simulink model "Ventilator_Controller"  (R2019b)
settings: Solver=ode23tb  StartTime=0  StopTime=1000  FixedStep=0.001  MaxStep=time_step_new  RelTol=0.01  EnableMultiTasking=on
values from neighbouring files (symbols this model uses):
  A = 20.9    [Gas_Exchange_IC.m]    (also in getPneumonia.m = (LF1-LF2)/(1-exp(Rresolve*(t2(end)-t2(1)))))
  a1 = 0.3836    [Dissociation_Spencer_IC.m]    (also in Gas_Exchange_IC.m; Respiratory_IC.m)
  a2 = 1.819    [Dissociation_Spencer_IC.m]    (also in Gas_Exchange_IC.m; Respiratory_IC.m)
  alpha1 = 0.02598    [Dissociation_Spencer_IC.m]    (also in Gas_Exchange_IC.m; Respiratory_IC.m)
  alpha2 = 0.05591    [Dissociation_Spencer_IC.m]    (also in Gas_Exchange_IC.m; Respiratory_IC.m)
  B = 92.8    [Gas_Exchange_IC.m]    (also in getPneumonia.m = LungFunction(end)-A)
  beta1 = 0.012275    [Dissociation_Spencer_IC.m]    (also in Gas_Exchange_IC.m; Respiratory_IC.m)
  beta2 = 0.03255    [Dissociation_Spencer_IC.m]    (also in Gas_Exchange_IC.m; Respiratory_IC.m)
  C = 10570    [Gas_Exchange_IC.m]
  C1 = 9    [Dissociation_Spencer_IC.m]    (also in Gas_Exchange_IC.m; Respiratory_IC.m)
  C2 = 87.00    (= 87)    [Dissociation_Spencer_IC.m]    (also in Gas_Exchange_IC.m; Respiratory_IC.m)
  Circadian_Period = 24    [Respiratory_IC.m]    (also in State_UA_Khoo_IC.m)
  CvCO2IC = 0.5116    [Body_Khoo_IC.m]    (also in Gas_Exchange_IC.m; Respiratory_IC.m = 0.5247)
  CvO2IC = 0.1672    [Body_Khoo_IC.m]    (also in Gas_Exchange_IC.m; Respiratory_IC.m = 0.1639)
  D = -5.251    [Gas_Exchange_IC.m]
  Dead1CO2IC = 0.1020    (= 0.102)    [Dead_Space_Khoo_IC.m]    (also in Gas_Exchange_IC.m; Respiratory_IC.m = 39.5616)
  Dead1O2IC = 149.8824    [Dead_Space_Khoo_IC.m]    (also in Gas_Exchange_IC.m; Respiratory_IC.m = 104.3637)
  Dead2CO2IC = 0.5274    [Dead_Space_Khoo_IC.m]    (also in Gas_Exchange_IC.m; Respiratory_IC.m = 39.6736)
  Dead2O2IC = 149.3923    [Dead_Space_Khoo_IC.m]    (also in Gas_Exchange_IC.m; Respiratory_IC.m = 104.2258)
  Dead3CO2IC = 2.2996    [Dead_Space_Khoo_IC.m]    (also in Gas_Exchange_IC.m; Respiratory_IC.m = 39.8127)
  Dead3O2IC = 147.3503    [Dead_Space_Khoo_IC.m]    (also in Gas_Exchange_IC.m; Respiratory_IC.m = 104.0505)
  Dead4CO2IC = 8.2293    [Dead_Space_Khoo_IC.m]    (also in Gas_Exchange_IC.m; Respiratory_IC.m = 40.0061)
  Dead4O2IC = 140.5179    [Dead_Space_Khoo_IC.m]    (also in Gas_Exchange_IC.m; Respiratory_IC.m = 103.8005)
  Dead5CO2IC = 22.0757    [Dead_Space_Khoo_IC.m]    (also in Gas_Exchange_IC.m; Respiratory_IC.m = 40.3359)
  Dead5O2IC = 124.5641    [Dead_Space_Khoo_IC.m]    (also in Gas_Exchange_IC.m; Respiratory_IC.m = 103.3579)
  DtotalIC = 0.3    [NeuroMuscular_IC.m]    (also in Respiratory_IC.m = 0.32)
  E_CW = 5    [Pleural_Schuessler_IC.m]    (also in Pmus_Flow_Younes_IC.m; Resp_Mech_IC.m; Respiratory_IC.m)
  E_L = 5    [Pleural_Schuessler_IC.m]    (also in Pmus_Flow_Younes_IC.m; Resp_Mech_IC.m; Respiratory_IC.m)
  fc = 0.4/60    (= 0.00666666666667)    [Respiratory_IC.m]    (also in State_UA_Khoo_IC.m)
  fcs_max = 47.78    [Cardiovascular_IC.m]    (also in Reflex_Ursino_IC.m)
  fcs_min = 2.52    [Cardiovascular_IC.m]    (also in Reflex_Ursino_IC.m)
  fcs_zero = 25    [Respiratory_IC.m]
  FlowIC = 0    [Pmus_Flow_Younes_IC.m]    (also in Resp_Mech_IC.m; Respiratory_IC.m)
  fp_inf = 6.3    [Respiratory_IC.m]
  fp_zero = 3.2    [Respiratory_IC.m]
  fs_inf = 2.10    (= 2.1)    [Respiratory_IC.m]
  fs_zero = 16.11    [Respiratory_IC.m]
  ftbs_min = 0.1    [Cardiovascular_IC.m]    (also in SA_Node_Ursino_IC.m)
  gc = 0.008/60    (= 0.000133333333333)    [Respiratory_IC.m]    (also in State_UA_Khoo_IC.m)
  h = 0.0183    [Brain_Khoo_IC.m]    (also in Gas_Exchange_IC.m; Respiratory_IC.m)
  HP_basal = 0.58    [Cardiovascular_IC.m]    (also in SA_Node_Ursino_IC.m)
  Ic = 45    [Gas_Exchange_IC.m]    (also in Respiratory_IC.m; Vent_Drive_Khoo_IC.m)
  IpCO2 = 38    [Gas_Exchange_IC.m]    (also in Respiratory_IC.m; Vent_Drive_Khoo_IC.m)
  IpO2 = 102.4    [Gas_Exchange_IC.m]    (also in Respiratory_IC.m; Vent_Drive_Khoo_IC.m)
  K1 = 13    [Dissociation_Spencer_IC.m]    (also in Gas_Exchange_IC.m; Respiratory_IC.m)
  K2 = 194.4    [Dissociation_Spencer_IC.m]    (also in Gas_Exchange_IC.m; Respiratory_IC.m)
  k_cs = 11.758    [Cardiovascular_IC.m]    (also in Reflex_Ursino_IC.m)
  k_p = 7.06    [Respiratory_IC.m]
  k_s = 0.07    [Respiratory_IC.m]
  lambda = 863    [Gas_Exchange_IC.m]    (also in Lungs_Khoo_IC.m; Respiratory_IC.m)
  Mech_Vent_pressure = 17    [Mech_vent_test.m]
  MRbCO2 = 0.0517    [Brain_Khoo_IC.m]    (also in Gas_Exchange_IC.m; Respiratory_IC.m)
  MRCO2 = 0.0033    [Body_Khoo_IC.m]    (also in Gas_Exchange_IC.m; Respiratory_IC.m)
  MRO2 = 0.0038    [Body_Khoo_IC.m]    (also in Gas_Exchange_IC.m; Respiratory_IC.m)
  NM_block_gain = 1    [Mech_vent_test.m]
  PACO2_delayIC = 39.6041    [Cardio_Mix_Lange_IC.m]    (also in Gas_Exchange_IC.m; Respiratory_IC.m = 40.4448)
  PaCO2firstIC = 0.2150    (= 0.215)    [Cardio_Mix_Lange_IC.m]    (also in Gas_Exchange_IC.m; Respiratory_IC.m = -0.2465)
  PACO2IC = 37.1484    [Gas_Exchange_IC.m]    (also in Lungs_Khoo_IC.m; Respiratory_IC.m = 40.9432)
  PaCO2secondIC = 38.4577    [Cardio_Mix_Lange_IC.m]    (also in Gas_Exchange_IC.m; Respiratory_IC.m = 40.3928)
  PAO2_delayIC = 103.8436    [Cardio_Mix_Lange_IC.m]    (also in Gas_Exchange_IC.m; Respiratory_IC.m = 103.1223)
  PaO2firstIC = -0.2838    [Cardio_Mix_Lange_IC.m]    (also in Gas_Exchange_IC.m; Respiratory_IC.m = 0.3557)
  PAO2IC = 107.1983    [Gas_Exchange_IC.m]    (also in Lungs_Khoo_IC.m; Respiratory_IC.m = 102.5153)
  PaO2secondIC = 105.4828    [Cardio_Mix_Lange_IC.m]    (also in Gas_Exchange_IC.m; Respiratory_IC.m = 103.1435)
  PbCO2IC = 48.2858    [Brain_Khoo_IC.m]    (also in Gas_Exchange_IC.m; Respiratory_IC.m = 48.5383)
  PICO2 = 0    [Dead_Space_Khoo_IC.m]    (also in Gas_Exchange_IC.m; Respiratory_IC.m)
  PICO2_change = 0    [Respiratory_IC.m]
  PIO2 = 150    [Dead_Space_Khoo_IC.m]    (also in Gas_Exchange_IC.m; Respiratory_IC.m)
  PIO2_change = -90    [Mech_vent_test.m]    (also in Respiratory_IC.m = 0)
  Pn = 90    [Cardiovascular_IC.m]    (also in Reflex_Ursino_IC.m)
  Pt_frcIC1 = 0    [Pmus_Flow_Younes_IC.m]    (also in Resp_Mech_IC.m; Respiratory_IC.m)
  Pt_frcIC2 = 0    [Pmus_Flow_Younes_IC.m]    (also in Resp_Mech_IC.m; Respiratory_IC.m)
  QdBo = 0.8333    [Brain_Khoo_IC.m]    (also in Gas_Exchange_IC.m; Respiratory_IC.m)
  R_AW = 1.27    [Pleural_Schuessler_IC.m]    (also in Pmus_Flow_Younes_IC.m; Resp_Mech_IC.m; Respiratory_IC.m)
  R_CW = 1.03    [Pleural_Schuessler_IC.m]    (also in Pmus_Flow_Younes_IC.m; Resp_Mech_IC.m; Respiratory_IC.m)
  R_L = 1.69    [Pleural_Schuessler_IC.m]    (also in Pmus_Flow_Younes_IC.m; Resp_Mech_IC.m; Respiratory_IC.m)
  RC = 0.06    [Pleural_Schuessler_IC.m]    (also in Pmus_Flow_Younes_IC.m; Resp_Mech_IC.m; Respiratory_IC.m)
  rc = 0.2/60    (= 0.00333333333333)    [Respiratory_IC.m]    (also in State_UA_Khoo_IC.m)
  SbCO2 = 0.3600    (= 0.36)    [Brain_Khoo_IC.m]    (also in Gas_Exchange_IC.m; Respiratory_IC.m)
  SCO2 = 0.0043    [Brain_Khoo_IC.m]    (also in Gas_Exchange_IC.m; Respiratory_IC.m)
  SWAo = 0.007    [Respiratory_IC.m]    (also in State_UA_Khoo_IC.m)
  T1 = 1    [Cardio_Mix_Lange_IC.m]    (also in Gas_Exchange_IC.m; Respiratory_IC.m)
  T2 = 2    [Cardio_Mix_Lange_IC.m]    (also in Gas_Exchange_IC.m; Respiratory_IC.m)
  t_CO2_duration = 0    [Respiratory_IC.m]
  t_CO2_start = 0    [Respiratory_IC.m]
  t_end_new = 4*24*60*60    (= 345600)    [Mech_vent_test.m]
  t_end_UA = 0    [Respiratory_IC.m]    (also in State_UA_Khoo_IC.m)
  t_Mech_Vent_duration = 0    [Mech_vent_test.m]
  t_Mech_Vent_start = 0    [Mech_vent_test.m]
  t_Mueller_duration = 0    [NeuroMuscular_IC.m]
  t_Mueller_insp = 0    [NeuroMuscular_IC.m]
  t_Mueller_start = 0    [NeuroMuscular_IC.m]
  t_NM_block_duration = 0    [Mech_vent_test.m]
  t_NM_block_start = 0    [Mech_vent_test.m]
  t_O2_duration = 0    [Mech_vent_test.m]    (also in Respiratory_IC.m)
  t_O2_start = 0    [Mech_vent_test.m]    (also in Respiratory_IC.m)
  t_start_new = 0    [Mech_vent_test.m]
  t_start_UA = 0    [Respiratory_IC.m]    (also in State_UA_Khoo_IC.m)
  t_valsalva_duration = 0    [NeuroMuscular_IC.m]
  t_valsalva_insp = 0    [NeuroMuscular_IC.m]
  t_valsalva_start = 0    [NeuroMuscular_IC.m]
  time_step = time_step    [acquire_data.m]    (also in acquire_data_save.m)
  VC = 5    [Pmus_Flow_Younes_IC.m]    (also in Resp_Mech_IC.m; Respiratory_IC.m)
  Vdead1 = 0.03    [Dead_Space_Khoo_IC.m]    (also in Gas_Exchange_IC.m; Respiratory_IC.m)
  Vdead2 = 0.03    [Dead_Space_Khoo_IC.m]    (also in Gas_Exchange_IC.m; Respiratory_IC.m)
  Vdead3 = 0.03    [Dead_Space_Khoo_IC.m]    (also in Gas_Exchange_IC.m; Respiratory_IC.m)
  Vdead4 = 0.03    [Dead_Space_Khoo_IC.m]    (also in Gas_Exchange_IC.m; Respiratory_IC.m)
  Vdead5 = 0.03    [Dead_Space_Khoo_IC.m]    (also in Gas_Exchange_IC.m; Respiratory_IC.m)
  Ventilator_rate = 12    [Mech_vent_test.m]
  VTCO2 = 15    [Body_Khoo_IC.m]    (also in Gas_Exchange_IC.m; Respiratory_IC.m)
  VtIC = 0    [Pmus_Flow_Younes_IC.m]    (also in Resp_Mech_IC.m; Respiratory_IC.m)
  VTO2 = 6    [Body_Khoo_IC.m]    (also in Gas_Exchange_IC.m; Respiratory_IC.m)
  Z = 0.0227    [Dissociation_Spencer_IC.m]    (also in Gas_Exchange_IC.m; Respiratory_IC.m)
undefined symbols (not defined in the file or in its folder): A_0_ua, alpha_E_FFA_Heart, alpha_E_FFA_muscle, alpha_E_GLC_Heart, alpha_E_GLC_muscle, alpha_E_GLY_muscle, alpha_E_PYR_muscle, alpha_E_TGL_adipose, alpha_E_TGL_GI, alpha_E_TGL_Heart, alpha_E_TGL_muscle, Arousal_UAIC, C_ua_awake, Cbp, Cbv, Ce_0, Cep, Cev, Chp, Chv, Cla, Clamp_class, Cmp, Cmv, Cpa, CPAP_pressure, Cpp, Cpv, Cra, Csa, Csp, Csv, CvbO2_n, CvhO2_n, CvmO2_n, DAY, delay, DietBlock, Dx, Fb, fchemo_max, fchemo_min, fchemoIC, flsIC, Ftas_I0, ftas_min, ftas_r0, FVC_activation, gain_E, Gamma, Gas_sleep, Gas_sleepM, Gb, Gblock, GbO2, Gbs_sleep, gcc_sa, gcc_sb, gcc_sp, Gclamp ... (+147)
libraries: simulink x4, simulink_extras x2
(part 4 of 8)

== system Ventilator_Controller/Cardiovascular System/SA-node and Autonomic Control/Heart Emaxrv ==
  ftbs : Inport
  Gbs(SI) : Inport  Port=2
  Constant : Constant  Value=ftbs_min
  Constant1 : Constant  Value=initx(2)
  Gain_Emaxrv : Gain  Gain=0.282  SaturateOnIntegerOverflow=on  OutDataTypeStr=Inherit: Same as input  ParamDataTypeStr=Inherit: Same as input
  Math Function : Math  Operator=log  SaturateOnIntegerOverflow=on
  Product3 : Product  SaturateOnIntegerOverflow=on  InputSameDT=on  OutDataTypeStr=Inherit: Same as first input
  Saturation : Saturate  UpperLimit=inf  LowerLimit=1
  Sum : Sum  Inputs=|+-  SaturateOnIntegerOverflow=on  InputSameDT=on  OutDataTypeStr=Inherit: Same as first input
  Sum1 : Sum  SaturateOnIntegerOverflow=on  InputSameDT=on  OutDataTypeStr=Inherit: Same as first input
  Transfer Fcn : TransferFcn  Denominator=[toux(2) 1]
  Transport Delay : TransportDelay  DelayTime=Dx(2)  BufferSize=19456
  Emaxrv : Outport
  wires:
  Constant1/1 -> Sum1/2
  Sum1/1 -> Emaxrv/1
  Transfer Fcn/1 -> Sum1/1
  Math Function/1 -> Gain_Emaxrv/1
  Saturation/1 -> Math Function/1
  Sum/1 -> Saturation/1
  Constant/1 -> Sum/2
  Transport Delay/1 -> Sum/1
  ftbs/1 -> Transport Delay/1
  Gbs(SI)/1 -> Product3/2
  Gain_Emaxrv/1 -> Product3/1
  Product3/1 -> Transfer Fcn/1

== system Ventilator_Controller/Cardiovascular System/SA-node and Autonomic Control/Hypoxia or hypercapnia1 ==
  Drive : Inport
  Divide : Product  Inputs=**
  Power : Outport
  wires:
  [MuscleContractility] -> Divide/1
  Divide/1 -> Power/1  "muscle power"
  Drive/1 -> Divide/2  "Muscle drive"

== system Ventilator_Controller/Cardiovascular System/SA-node and Autonomic Control/Hypoxia or hypercapnia2 ==
  Drive : Inport
  Divide : Product  Inputs=**
  Power : Outport
  wires:
  [MuscleContractility] -> Divide/1
  Divide/1 -> Power/1  "muscle power"
  Drive/1 -> Divide/2  "Muscle drive"

== system Ventilator_Controller/Cardiovascular System/SA-node and Autonomic Control/Left Ventricle ==
  phi : Inport
  Constant13 : Constant  Value=Vulv
  Constant14 : Constant  Value=P0lv
  Constant6 : Constant
  Fcn : Fcn  Expr=exp(u*KElv)-1
  Product4 : Product  Inputs=3  SaturateOnIntegerOverflow=on  RndMeth=Zero  InputSameDT=on  OutDataTypeStr=Inherit: Same as first input
  Product5 : Product  Inputs=3  SaturateOnIntegerOverflow=on  RndMeth=Zero  InputSameDT=on  OutDataTypeStr=Inherit: Same as first input
  SubSystem1 : Subsystem
  Sum2 : Sum  SaturateOnIntegerOverflow=on  InputSameDT=on  OutDataTypeStr=Inherit: Same as first input
  Sum3 : Sum  Inputs=-+  SaturateOnIntegerOverflow=on  InputSameDT=on  OutDataTypeStr=Inherit: Same as first input
  Pmaxlv : Outport
  wires:
  Sum2/1 -> Pmaxlv/1
  Product4/1 -> Sum2/1
  Product5/1 -> Sum2/2
  Fcn/1 -> Product5/1
  Constant14/1 -> Product5/2
  Sum3/1 -> Product5/3
  Constant6/1 -> Sum3/2
  Constant13/1 -> SubSystem1/1(_)
  [Vlv] -> SubSystem1/2(+)
  SubSystem1/1(Out) -> Product4/2
  phi/1 -> Sum3/1, Product4/3
  [Emaxlv] -> Product4/1
  [Vlv] -> Fcn/1

== system Ventilator_Controller/Cardiovascular System/SA-node and Autonomic Control/RR Interval ==
  HP_SAnode : Inport
  Abs : Abs  SaturateOnIntegerOverflow=on
  Derivative1 : Derivative
  If : If  IfExpression=u1 <0  ShowElse=off
  If Action Subsystem : Subsystem  TreatAsAtomicUnit=on
  Integrator : Integrator  ExternalReset=rising  UpperSaturationLimit=10  LowerSaturationLimit=0
  Integrator1 : Integrator  ExternalReset=rising  UpperSaturationLimit=10  LowerSaturationLimit=0
  Math Function : Math  Operator=reciprocal  SaturateOnIntegerOverflow=on
  Memory : Memory
  Mux : Mux
  Saving varHeartPeriod : Subsystem
  Sign1 : Signum  ZeroCross=off
  Sum : Sum  Inputs=+-  SaturateOnIntegerOverflow=on
  Threshold Integrated HP : Constant
  Time Constant : Constant
  Heart_Period : Outport
  wires:
  Threshold Integrated HP/1 -> Sum/1
  Integrator/1 -> Sum/2
  Sum/1 -> If/1, Mux/2  "HPin"
  Memory/1 -> Integrator/2, Integrator1/2
  Sign1/1 -> Abs/1
  Derivative1/1 -> Sign1/1
  Abs/1 -> Memory/1  "Enable signal"
  HP_SAnode/1 -> Math Function/1
  Time Constant/1 -> Integrator1/1
  Integrator1/1 -> If Action Subsystem/1(In1), Mux/3  "HPout"
  If Action Subsystem/1(Out1) -> Derivative1/1, Heart_Period/1, Mux/4  "Heart Period"
  If/1 -> If Action Subsystem/Action
  Math Function/1 -> Integrator/1, Mux/1
  Mux/1 -> Saving varHeartPeriod/1(In1)

== system Ventilator_Controller/Cardiovascular System/SA-node and Autonomic Control/Right Ventricle ==
  phi : Inport
  Constant13 : Constant  Value=Vurv
  Constant14 : Constant  Value=P0rv
  Constant6 : Constant
  Fcn : Fcn  Expr=exp(u*KErv)-1
  Product4 : Product  Inputs=3  SaturateOnIntegerOverflow=on  RndMeth=Zero  InputSameDT=on  OutDataTypeStr=Inherit: Same as first input
  Product5 : Product  Inputs=3  SaturateOnIntegerOverflow=on  RndMeth=Zero  InputSameDT=on  OutDataTypeStr=Inherit: Same as first input
  SubSystem1 : Subsystem
  Sum2 : Sum  SaturateOnIntegerOverflow=on  InputSameDT=on  OutDataTypeStr=Inherit: Same as first input
  Sum3 : Sum  Inputs=-+  SaturateOnIntegerOverflow=on  InputSameDT=on  OutDataTypeStr=Inherit: Same as first input
  Pmaxrv : Outport
  wires:
  Constant6/1 -> Sum3/2
  Sum3/1 -> Product5/3
  Constant14/1 -> Product5/2
  Fcn/1 -> Product5/1
  Product5/1 -> Sum2/2
  Product4/1 -> Sum2/1
  Sum2/1 -> Pmaxrv/1
  [Emaxrv] -> Product4/1
  [Vrv] -> SubSystem1/2(+)
  Constant13/1 -> SubSystem1/1(_)
  SubSystem1/1(Out) -> Product4/2
  phi/1 -> Sum3/1, Product4/3
  [Vrv] -> Fcn/1

== system Ventilator_Controller/Cardiovascular System/SA-node and Autonomic Control/SA Node ==
  ftbs : Inport
  ftp : Inport  Port=2
  Gbs(SI) : Inport  Port=3
  Gps(SI) : Inport  Port=4
  Constant : Constant  Value=ftbs_min
  Constant1 : Constant  Value=HP_basal
  Gain_HPbs : Gain  Gain=-0.13  SaturateOnIntegerOverflow=on  OutDataTypeStr=Inherit: Same as input  ParamDataTypeStr=Inherit: Same as input
  Gain_HPpara : Gain  Gain=0.09  SaturateOnIntegerOverflow=on  OutDataTypeStr=Inherit: Same as input  ParamDataTypeStr=Inherit: Same as input
  Math Function : Math  Operator=log  SaturateOnIntegerOverflow=on
  Product1 : Product  Inputs=*/  SaturateOnIntegerOverflow=on  InputSameDT=on  OutDataTypeStr=Inherit: Same as first input
  Product3 : Product  SaturateOnIntegerOverflow=on  InputSameDT=on  OutDataTypeStr=Inherit: Same as first input
  Saturation : Saturate  UpperLimit=inf  LowerLimit=1
  Sum : Sum  Inputs=+-  SaturateOnIntegerOverflow=on  InputSameDT=on  OutDataTypeStr=Inherit: Same as first input
  Sum1 : Sum  Inputs=+++  SaturateOnIntegerOverflow=on  InputSameDT=on  OutDataTypeStr=Inherit: Same as first input
  Transfer Fcn : TransferFcn  Denominator=[toux(7) 1]
  Transfer Fcn1 : TransferFcn  Denominator=[toux(8) 1]
  Transport Delay : TransportDelay  DelayTime=Dx(7)  BufferSize=19456
  Transport Delay1 : TransportDelay  DelayTime=Dx(8)  BufferSize=18432
  HP : Outport
  wires:
  ftbs/1 -> Transport Delay/1
  Transport Delay/1 -> Sum/1
  Constant/1 -> Sum/2
  Sum/1 -> Saturation/1
  Saturation/1 -> Math Function/1
  Math Function/1 -> Product3/2
  Gain_HPbs/1 -> Transfer Fcn/1
  Transfer Fcn/1 -> Sum1/1
  Sum1/1 -> HP/1
  Constant1/1 -> Sum1/2
  ftp/1 -> Transport Delay1/1
  Transport Delay1/1 -> Product1/1
  Gain_HPpara/1 -> Transfer Fcn1/1
  Transfer Fcn1/1 -> Sum1/3
  Gbs(SI)/1 -> Product3/1
  Product3/1 -> Gain_HPbs/1
  Product1/1 -> Gain_HPpara/1
  Gps(SI)/1 -> Product1/2

== system Ventilator_Controller/Cardiovascular System/SA-node and Autonomic Control/phi ==
  HP : Inport
  Constant3 : Constant  Value=0
  Constant4 : Constant  Value=ksys
  Constant5 : Constant  Value=Tsys0
  Constant6 : Constant
  Data Store Memory : DataStoreMemory  InitialValue=initx(7)  ShowAdditionalParam=off
  Data Store Read : DataStoreRead  SampleTime=0
  Fcn1 : Fcn  Expr=sin(pi*u)^2
  Integrator : Integrator
  Math Function2 : Math  Operator=rem  SaturateOnIntegerOverflow=on
  Math Function3 : Math  Operator=reciprocal  SaturateOnIntegerOverflow=on
  Product : Product  SaturateOnIntegerOverflow=on  RndMeth=Zero  InputSameDT=on  OutDataTypeStr=Inherit: Same as first input
  Product2 : Product  Inputs=/*  SaturateOnIntegerOverflow=on  RndMeth=Zero  InputSameDT=on  OutDataTypeStr=Inherit: Same as first input
  Product3 : Product  Inputs=*/  SaturateOnIntegerOverflow=on  RndMeth=Zero  InputSameDT=on  OutDataTypeStr=Inherit: Same as first input
  SubSystem : Subsystem  TreatAsAtomicUnit=on
  Sum1 : Sum  Inputs=-+  SaturateOnIntegerOverflow=on  InputSameDT=on  OutDataTypeStr=Inherit: Same as first input
  Switch : Switch  Threshold=1  SaturateOnIntegerOverflow=on  InputSameDT=on
  phi : Outport
  wires:
  Product3/1 -> Product/2
  Sum1/1 -> Product3/2
  Constant5/1 -> Sum1/2
  Product2/1 -> Sum1/1
  Constant4/1 -> Product2/2
  Constant3/1 -> Switch/1
  Product/1 -> Switch/2, Switch/3
  Fcn1/1 -> phi/1
  HP/1 -> SubSystem/1(In1)  "heart period"
  Switch/1 -> Fcn1/1, SubSystem/Trigger
  Data Store Read/1 -> Product3/1, Product2/1, Math Function3/1  "heart period"
  Constant6/1 -> Math Function2/2
  Math Function2/1 -> Product/1  "u"
  Math Function3/1 -> Integrator/1
  Integrator/1 -> Math Function2/1

== system Ventilator_Controller/Cardiovascular System/Systemic/Systemic Arteries ==
  Qlv : Inport
  Constant2 : Constant  Value=Vusa
  Gain : Gain  Gain=1/Csa  SaturateOnIntegerOverflow=on  OutDataTypeStr=Inherit: Same as input  ParamDataTypeStr=Inherit: Same as input
  Gain1 : Gain  Gain=1/Lsa  SaturateOnIntegerOverflow=on  OutDataTypeStr=Inherit: Same as input  ParamDataTypeStr=Inherit: Same as input
  Gain2 : Gain  Gain=Rsa  SaturateOnIntegerOverflow=on  OutDataTypeStr=Inherit: Same as input  ParamDataTypeStr=Inherit: Same as input
  Integrator : Integrator  InitialCondition=25.863
  Integrator1 : Integrator
  SubSystem : Subsystem
  Sum : Sum  Inputs=|+-
  Sum1 : Sum  Inputs=+-  SaturateOnIntegerOverflow=on  InputSameDT=on  OutDataTypeStr=Inherit: Same as first input
  Sum2 : Sum  Inputs=-+-  SaturateOnIntegerOverflow=on  InputSameDT=on  OutDataTypeStr=Inherit: Same as first input
  Qsa : Outport
  tag scope: ABP=global, Vsa=scoped
  wires:
  Sum1/1 -> Integrator/1
  Integrator1/1 -> Gain1/1
  Sum2/1 -> Integrator1/1
  Gain2/1 -> Sum2/3
  Gain1/1 -> Sum1/2, Gain2/1, Qsa/1  "Qsa"
  Integrator/1 -> SubSystem/2(+)
  SubSystem/1(Out) -> Gain/1, [Vsa]
  Constant2/1 -> SubSystem/1(_)
  Qlv/1 -> Sum1/1
  [Psp] -> Sum2/1
  [gPpl] -> Sum/2
  Gain/1 -> Sum/1, [ABP]  "Psa"
  Sum/1 -> Sum2/2

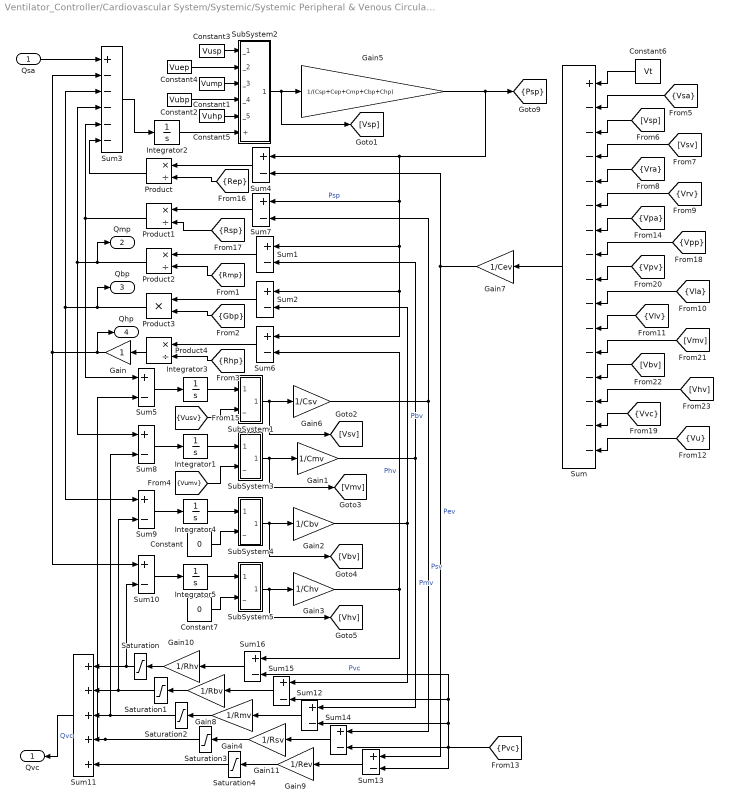
== system Ventilator_Controller/Cardiovascular System/Systemic/Systemic Peripheral & Venous Circulation ==
  Qsa : Inport
  Constant : Constant  Value=0
  Constant1 : Constant  Value=Vump
  Constant2 : Constant  Value=Vubp
  Constant3 : Constant  Value=Vusp
  Constant4 : Constant  Value=Vuep
  Constant5 : Constant  Value=Vuhp
  Constant6 : Constant  Value=Vt
  Constant7 : Constant  Value=0
  Gain : Gain
  Gain1 : Gain  Gain=1/Cmv  SaturateOnIntegerOverflow=on  OutDataTypeStr=Inherit: Same as input  ParamDataTypeStr=Inherit: Same as input
  Gain10 : Gain  Gain=1/Rhv  SaturateOnIntegerOverflow=on  OutDataTypeStr=Inherit: Same as input  ParamDataTypeStr=Inherit: Same as input
  Gain11 : Gain  Gain=1/Rsv  SaturateOnIntegerOverflow=on  OutDataTypeStr=Inherit: Same as input  ParamDataTypeStr=Inherit: Same as input
  Gain2 : Gain  Gain=1/Cbv  SaturateOnIntegerOverflow=on  OutDataTypeStr=Inherit: Same as input  ParamDataTypeStr=Inherit: Same as input
  Gain3 : Gain  Gain=1/Chv  SaturateOnIntegerOverflow=on  OutDataTypeStr=Inherit: Same as input  ParamDataTypeStr=Inherit: Same as input
  Gain4 : Gain  Gain=1/Rmv  SaturateOnIntegerOverflow=on  OutDataTypeStr=Inherit: Same as input  ParamDataTypeStr=Inherit: Same as input
  Gain5 : Gain  Gain=1/(Csp+Cep+Cmp+Cbp+Chp)  SaturateOnIntegerOverflow=on  OutDataTypeStr=Inherit: Same as input  ParamDataTypeStr=Inherit: Same as input
  Gain6 : Gain  Gain=1/Csv  SaturateOnIntegerOverflow=on  OutDataTypeStr=Inherit: Same as input  ParamDataTypeStr=Inherit: Same as input
  Gain7 : Gain  Gain=1/Cev  SaturateOnIntegerOverflow=on  OutDataTypeStr=Inherit: Same as input  ParamDataTypeStr=Inherit: Same as input
  Gain8 : Gain  Gain=1/Rbv  SaturateOnIntegerOverflow=on  OutDataTypeStr=Inherit: Same as input  ParamDataTypeStr=Inherit: Same as input
  Gain9 : Gain  Gain=1/Rev  SaturateOnIntegerOverflow=on  OutDataTypeStr=Inherit: Same as input  ParamDataTypeStr=Inherit: Same as input
  Integrator{1,3..5} (4 alike) : Integrator
  Integrator2 : Integrator  InitialCondition=Vusp + Vuep+Vump+Vubp+Vuhp
  Product{,1..2,4} (4 alike) : Product  Inputs=*/  SaturateOnIntegerOverflow=on  RndMeth=Zero  InputSameDT=on  OutDataTypeStr=Inherit: Same as first input
  Product3 : Product  Inputs=**  SaturateOnIntegerOverflow=on  RndMeth=Zero  InputSameDT=on  OutDataTypeStr=Inherit: Same as first input
  Saturation : Saturate  UpperLimit=10000  LowerLimit=1
  Saturation1 : Saturate  UpperLimit=10000  LowerLimit=4
  Saturation2 : Saturate  UpperLimit=10000  LowerLimit=8
  Saturation3 : Saturate  UpperLimit=10000  LowerLimit=10
  Saturation4 : Saturate  UpperLimit=10000  LowerLimit=10
  SubSystem1 : Subsystem
  SubSystem2 : Subsystem
  SubSystem3 : Subsystem
  SubSystem4 : Subsystem
  SubSystem5 : Subsystem
  Sum : Sum  Inputs=+---------------  SaturateOnIntegerOverflow=on  InputSameDT=on  OutDataTypeStr=Inherit: Same as first input
  Sum{1..2,4..10,12..16} (14 alike) : Sum  Inputs=+-  SaturateOnIntegerOverflow=on  InputSameDT=on  OutDataTypeStr=Inherit: Same as first input
  Sum11 : Sum  Inputs=+++++  SaturateOnIntegerOverflow=on  InputSameDT=on  OutDataTypeStr=Inherit: Same as first input
  Sum3 : Sum  Inputs=+-----  SaturateOnIntegerOverflow=on  InputSameDT=on  OutDataTypeStr=Inherit: Same as first input
  Qvc : Outport
  Qmp : Outport  Port=2
  Qbp : Outport  Port=3
  Qhp : Outport  Port=4
  tag scope: Psp=scoped
  wires:
  Gain5/1 -> Sum4/1, Sum6/1, Sum2/1, Sum1/1, Sum7/1, [Psp]  "Psp"
  Product1/1 -> Sum3/5, Sum5/1
  Integrator3/1 -> SubSystem1/1(+)
  SubSystem1/1(Out) -> Gain6/1, [Vsv]
  Integrator2/1 -> SubSystem2/6(+)
  SubSystem2/1(Out) -> Gain5/1, [Vsp]
  Sum13/1 -> Gain9/1
  Gain9/1 -> Saturation4/1
  Sum14/1 -> Gain11/1
  [Pvc] -> Sum13/2, Sum14/2, Sum12/2, Sum15/2, Sum16/2  "Pvc"
  Sum5/1 -> Integrator3/1
  Gain11/1 -> Saturation3/1
  [Vusv] -> SubSystem1/2(_)
  Constant3/1 -> SubSystem2/1(_1)
  Constant4/1 -> SubSystem2/2(_2)
  Sum4/1 -> Product/1
  [Rep] -> Product/2
  [Rsp] -> Product1/2
  Sum7/1 -> Product1/1
  Gain6/1 -> Sum7/2, Sum14/1  "Psv"
  Qsa/1 -> Sum3/1
  Gain7/1 -> Sum4/2, Sum13/1  "Pev"
  Sum11/1 -> Qvc/1  "Qvc"
  Sum1/1 -> Product2/1
  [Rmp] -> Product2/2
  Sum2/1 -> Product3/1
  [Gbp] -> Product3/2
  Sum6/1 -> Product4/1
  [Rhp] -> Product4/2
  Product4/1 -> Gain/1
  Product3/1 -> Sum3/3, Sum9/1, Qbp/1
  Product2/1 -> Sum3/4, Sum8/1, Qmp/1
  Product/1 -> Sum3/6
  Constant1/1 -> SubSystem2/3(_3)
  Constant2/1 -> SubSystem2/4(_4)
  Constant5/1 -> SubSystem2/5(_5)
  Sum3/1 -> Integrator2/1
  Integrator1/1 -> SubSystem3/1(+)
  SubSystem3/1(Out) -> Gain1/1, [Vmv]
  Sum8/1 -> Integrator1/1
  [Vumv] -> SubSystem3/2(_)
  Constant6/1 -> Sum/1
  [Vsa] -> Sum/2
  [Vsp] -> Sum/3
  [Vsv] -> Sum/4
  [Vra] -> Sum/5
  [Vrv] -> Sum/6
  [Vpa] -> Sum/7
  [Vpp] -> Sum/8
  [Vpv] -> Sum/9
  [Vla] -> Sum/10
  [Vlv] -> Sum/11
  [Vu] -> Sum/16
  [Vvc] -> Sum/15
  Sum/1 -> Gain7/1
  [Vmv] -> Sum/12
  [Vbv] -> Sum/13
  [Vhv] -> Sum/14
  Integrator4/1 -> SubSystem4/1(+)
  SubSystem4/1(Out) -> Gain2/1, [Vbv]
  Sum9/1 -> Integrator4/1
  Constant/1 -> SubSystem4/2(_)
  Integrator5/1 -> SubSystem5/1(+)
  SubSystem5/1(Out) -> Gain3/1, [Vhv]
  Sum10/1 -> Integrator5/1
  Constant7/1 -> SubSystem5/2(_)
  Gain1/1 -> Sum1/2, Sum12/1  "Pmv"
  Gain2/1 -> Sum2/2, Sum15/1  "Pbv"
  Gain3/1 -> Sum6/2, Sum16/1  "Phv"
  Sum12/1 -> Gain4/1
  Gain4/1 -> Saturation2/1
  Sum15/1 -> Gain8/1
  Gain8/1 -> Saturation1/1
  Sum16/1 -> Gain10/1
  Gain10/1 -> Saturation/1
  Gain/1 -> Sum3/2, Sum10/1, Qhp/1
  Saturation/1 -> Sum11/1, Sum10/2
  Saturation1/1 -> Sum11/2, Sum9/2
  Saturation2/1 -> Sum11/3, Sum8/2
  Saturation3/1 -> Sum5/2, Sum11/4
  Saturation4/1 -> Sum11/5

== system Ventilator_Controller/Cardiovascular System/Systemic/Vena Cava ==
  Qvc : Inport
  Integrator4 : Integrator
  Product2 : Product  Inputs=*/  SaturateOnIntegerOverflow=on  RndMeth=Zero  InputSameDT=on  OutDataTypeStr=Inherit: Same as first input
  Pvc : Fcn  Expr=(u>=V_vc_0)*(D1+K1_vc*(u-V_vc_0)) + ( u<V_vc_0)*(D2 + K2_vc*exp(u/V_vc_min))
  Rvc : Fcn  Expr="Kr_vc * (V_vc_max/u)*  (V_vc_max/u) + R_vc_0"
  Saturation : Saturate  UpperLimit=10000  LowerLimit=0  ZeroCross=off
  SubSystem3 : Subsystem
  Sum10 : Sum  Inputs=+-  SaturateOnIntegerOverflow=on  InputSameDT=on  OutDataTypeStr=Inherit: Same as first input
  Sum12 : Sum  Inputs=+-  SaturateOnIntegerOverflow=on  InputSameDT=on  OutDataTypeStr=Inherit: Same as first input
  Sum8 : Sum  Inputs=|++
  V_vc_0 : Constant  Value=130
  Qra : Outport
  tag scope: Pvc=scoped, Vvc=scoped
  wires:
  [gPpl] -> Sum8/2
  Integrator4/1 -> SubSystem3/1(+)
  Sum10/1 -> Integrator4/1
  V_vc_0/1 -> SubSystem3/2(_)
  Pvc/1 -> Sum8/1
  SubSystem3/1(Out) -> Pvc/1, [Vvc]
  Sum8/1 -> [Pvc], Sum12/1
  [Vvc] -> Rvc/1
  [Pra] -> Sum12/2
  Sum12/1 -> Product2/1
  Rvc/1 -> Product2/2
  Product2/1 -> Saturation/1  "Qra"
  Qvc/1 -> Sum10/1
  Saturation/1 -> Sum10/2, Qra/1

== system Ventilator_Controller/Cardiovascular System/TPR Change/Peri Circ Rep ==
  fes : Inport
  Gas(SI) : Inport  Port=2
  Constant : Constant  Value=ftas_min
  Constant1 : Constant  Value=initx(4)
  Gain1 : Gain  Gain=0.5  SaturateOnIntegerOverflow=on  OutDataTypeStr=Inherit: Same as input  ParamDataTypeStr=Inherit: Same as input
  Gain_Rep : Gain  Gain=1.94  SaturateOnIntegerOverflow=on  OutDataTypeStr=Inherit: Same as input  ParamDataTypeStr=Inherit: Same as input
  Math Function : Math  Operator=log  SaturateOnIntegerOverflow=on
  Product3 : Product  SaturateOnIntegerOverflow=on  InputSameDT=on  OutDataTypeStr=Inherit: Same as first input
  Saturation : Saturate  UpperLimit=inf  LowerLimit=1
  Sum : Sum  Inputs=|+-  SaturateOnIntegerOverflow=on  InputSameDT=on  OutDataTypeStr=Inherit: Same as first input
  Sum1 : Sum  SaturateOnIntegerOverflow=on  InputSameDT=on  OutDataTypeStr=Inherit: Same as first input
  Transfer Fcn : TransferFcn  Denominator=[toux(4) 1]
  Transport Delay : TransportDelay  DelayTime=Dx(4)*0.7  InitialOutput=10  BufferSize=19456
  Rep : Outport
  wires:
  Constant1/1 -> Gain1/1
  Sum1/1 -> Rep/1
  Transfer Fcn/1 -> Sum1/1
  Math Function/1 -> Gain_Rep/1
  Saturation/1 -> Math Function/1
  Sum/1 -> Saturation/1
  Constant/1 -> Sum/2
  Transport Delay/1 -> Sum/1
  fes/1 -> Transport Delay/1
  Gas(SI)/1 -> Product3/2
  Gain_Rep/1 -> Product3/1
  Product3/1 -> Transfer Fcn/1
  Gain1/1 -> Sum1/2

== system Ventilator_Controller/Cardiovascular System/TPR Change/Peri Circ Rmp ==
  fes : Inport
  Gas(SI) : Inport  Port=2
  Constant : Constant  Value=ftas_min
  Constant1 : Constant  Value=initx(10)
  Gain1 : Gain  Gain=0.5  SaturateOnIntegerOverflow=on  OutDataTypeStr=Inherit: Same as input  ParamDataTypeStr=Inherit: Same as input
  Gain_Rmp : Gain  Gain=2.47  SaturateOnIntegerOverflow=on  OutDataTypeStr=Inherit: Same as input  ParamDataTypeStr=Inherit: Same as input
  Math Function : Math  Operator=log  SaturateOnIntegerOverflow=on
  Product3 : Product  SaturateOnIntegerOverflow=on  InputSameDT=on  OutDataTypeStr=Inherit: Same as first input
  Saturation : Saturate  UpperLimit=inf  LowerLimit=1
  Sum : Sum  Inputs=+-  SaturateOnIntegerOverflow=on  InputSameDT=on  OutDataTypeStr=Inherit: Same as first input
  Sum1 : Sum  SaturateOnIntegerOverflow=on  InputSameDT=on  OutDataTypeStr=Inherit: Same as first input
  Transfer Fcn : TransferFcn  Denominator=[toux(10) 1]
  Transport Delay : TransportDelay  DelayTime=Dx(10)*0.7  InitialOutput=10  BufferSize=19456
  Rmp_n : Outport
  wires:
  Constant1/1 -> Gain1/1
  Sum1/1 -> Rmp_n/1
  Transfer Fcn/1 -> Sum1/1
  Math Function/1 -> Gain_Rmp/1
  Saturation/1 -> Math Function/1
  Sum/1 -> Saturation/1
  Constant/1 -> Sum/2
  Transport Delay/1 -> Sum/1
  fes/1 -> Transport Delay/1
  Gas(SI)/1 -> Product3/2
  Gain_Rmp/1 -> Product3/1
  Product3/1 -> Transfer Fcn/1
  Gain1/1 -> Sum1/2

== system Ventilator_Controller/Cardiovascular System/TPR Change/Peri Circ Rsp ==
  fes : Inport
  Gas(SI) : Inport  Port=2
  Constant : Constant  Value=ftas_min
  Constant1 : Constant  Value=initx(3)
  Gain : Gain  Gain=0.5  SaturateOnIntegerOverflow=on  OutDataTypeStr=Inherit: Same as input  ParamDataTypeStr=Inherit: Same as input
  Gain_Rsp : Gain  Gain=0.695  SaturateOnIntegerOverflow=on  OutDataTypeStr=Inherit: Same as input  ParamDataTypeStr=Inherit: Same as input
  Math Function : Math  Operator=log  SaturateOnIntegerOverflow=on
  Product3 : Product  SaturateOnIntegerOverflow=on  InputSameDT=on  OutDataTypeStr=Inherit: Same as first input
  Saturation : Saturate  UpperLimit=inf  LowerLimit=1
  Sum : Sum  Inputs=+-  SaturateOnIntegerOverflow=on  InputSameDT=on  OutDataTypeStr=Inherit: Same as first input
  Sum1 : Sum  SaturateOnIntegerOverflow=on  InputSameDT=on  OutDataTypeStr=Inherit: Same as first input
  Transfer Fcn : TransferFcn  Denominator=[toux(3) 1]
  Transport Delay : TransportDelay  DelayTime=Dx(3)*0.7  InitialOutput=10  BufferSize=19456
  Rsp : Outport
  wires:
  fes/1 -> Transport Delay/1
  Transport Delay/1 -> Sum/1
  Constant/1 -> Sum/2
  Sum/1 -> Saturation/1
  Saturation/1 -> Math Function/1
  Math Function/1 -> Gain_Rsp/1
  Transfer Fcn/1 -> Sum1/1
  Sum1/1 -> Rsp/1
  Constant1/1 -> Gain/1
  Gas(SI)/1 -> Product3/2
  Gain_Rsp/1 -> Product3/1
  Product3/1 -> Transfer Fcn/1
  Gain/1 -> Sum1/2

== system Ventilator_Controller/Cardiovascular System/TPR Change/Saving TPR ==
  In1 : Inport
  Clock : Clock
  Gain : Gain  Gain=1/(3600*24*7)
  Rounding Function : Rounding
  Switch Case : SwitchCase  CaseConditions={0,1,2,3,4,5,6,7,8}  SampleTime=0.1
  Switch Case Action Subsystem : Subsystem  TreatAsAtomicUnit=on
  Switch Case Action Subsystem1 : Subsystem  TreatAsAtomicUnit=on
  Switch Case Action Subsystem2 : Subsystem  TreatAsAtomicUnit=on
  Switch Case Action Subsystem3 : Subsystem  TreatAsAtomicUnit=on
  Switch Case Action Subsystem4 : Subsystem  TreatAsAtomicUnit=on
  Switch Case Action Subsystem5 : Subsystem  TreatAsAtomicUnit=on
  Switch Case Action Subsystem6 : Subsystem  TreatAsAtomicUnit=on
  Switch Case Action Subsystem7 : Subsystem  TreatAsAtomicUnit=on
  Switch Case Action Subsystem8 : Subsystem  TreatAsAtomicUnit=on
  Switch Case Action Subsystem9 : Subsystem  TreatAsAtomicUnit=on
  wires:
  Clock/1 -> Gain/1
  Switch Case/1 -> Switch Case Action Subsystem/Action
  Switch Case/2 -> Switch Case Action Subsystem1/Action
  Switch Case/3 -> Switch Case Action Subsystem2/Action
  Switch Case/10 -> Switch Case Action Subsystem3/Action
  Rounding Function/1 -> Switch Case/1
  In1/1 -> Switch Case Action Subsystem/1(In1), Switch Case Action Subsystem1/1(In1), Switch Case Action Subsystem2/1(In1), Switch Case Action Subsystem5/1(In1), Switch Case Action Subsystem3/1(In1), Switch Case Action Subsystem9/1(In1), Switch Case Action Subsystem8/1(In1), Switch Case Action Subsystem7/1(In1), Switch Case Action Subsystem6/1(In1), Switch Case Action Subsystem4/1(In1)
  Gain/1 -> Rounding Function/1
  Switch Case/4 -> Switch Case Action Subsystem4/Action
  Switch Case/5 -> Switch Case Action Subsystem5/Action
  Switch Case/6 -> Switch Case Action Subsystem6/Action
  Switch Case/7 -> Switch Case Action Subsystem7/Action
  Switch Case/8 -> Switch Case Action Subsystem8/Action
  Switch Case/9 -> Switch Case Action Subsystem9/Action

== system Ventilator_Controller/Cardiovascular System/TPR Change/Venous Circ Vuev ==
  fes : Inport
  Gas(SI) : Inport  Port=2
  Constant : Constant  Value=ftas_min
  Constant1 : Constant  Value=initx(6)
  Divide : Product  Inputs=**
  Gain_Vuev : Gain  Gain=-74.21  SaturateOnIntegerOverflow=on  OutDataTypeStr=Inherit: Same as input  ParamDataTypeStr=Inherit: Same as input
  Math Function : Math  Operator=log  SaturateOnIntegerOverflow=on
  Saturation : Saturate  UpperLimit=inf  LowerLimit=1
  Sum : Sum  Inputs=|+-  SaturateOnIntegerOverflow=on  InputSameDT=on  OutDataTypeStr=Inherit: Same as first input
  Sum1 : Sum  SaturateOnIntegerOverflow=on  InputSameDT=on  OutDataTypeStr=Inherit: Same as first input
  Transfer Fcn : TransferFcn  Denominator=[toux(6)*0.7 1]
  Transport Delay : TransportDelay  DelayTime=Dx(6)*0.7  InitialOutput=10  BufferSize=19456
  Vuev : Outport
  wires:
  Constant1/1 -> Sum1/2
  Sum1/1 -> Vuev/1
  Transfer Fcn/1 -> Sum1/1
  Math Function/1 -> Gain_Vuev/1
  Saturation/1 -> Math Function/1
  Sum/1 -> Saturation/1
  Constant/1 -> Sum/2
  Transport Delay/1 -> Sum/1
  fes/1 -> Transport Delay/1
  Gain_Vuev/1 -> Divide/1
  Divide/1 -> Transfer Fcn/1
  Gas(SI)/1 -> Divide/2

== system Ventilator_Controller/Cardiovascular System/TPR Change/Venous Circ Vumv ==
  fes : Inport
  Gas(SI) : Inport  Port=2
  Constant : Constant  Value=ftas_min
  Constant1 : Constant  Value=initx(9)
  Divide : Product  Inputs=**
  Gain_Vumv : Gain  Gain=-58.29  SaturateOnIntegerOverflow=on  OutDataTypeStr=Inherit: Same as input  ParamDataTypeStr=Inherit: Same as input
  Math Function : Math  Operator=log  SaturateOnIntegerOverflow=on
  Saturation : Saturate  UpperLimit=inf  LowerLimit=1
  Sum : Sum  Inputs=+-  SaturateOnIntegerOverflow=on  InputSameDT=on  OutDataTypeStr=Inherit: Same as first input
  Sum1 : Sum  SaturateOnIntegerOverflow=on  InputSameDT=on  OutDataTypeStr=Inherit: Same as first input
  Transfer Fcn : TransferFcn  Denominator=[toux(9)*0.7 1]
  Transport Delay : TransportDelay  DelayTime=Dx(9)*0.7  InitialOutput=10  BufferSize=19456
  Vumv : Outport
  wires:
  Constant1/1 -> Sum1/2
  Sum1/1 -> Vumv/1
  Transfer Fcn/1 -> Sum1/1
  Math Function/1 -> Gain_Vumv/1
  Saturation/1 -> Math Function/1
  Sum/1 -> Saturation/1
  Constant/1 -> Sum/2
  Transport Delay/1 -> Sum/1
  fes/1 -> Transport Delay/1
  Gas(SI)/1 -> Divide/2
  Gain_Vumv/1 -> Divide/1
  Divide/1 -> Transfer Fcn/1

== system Ventilator_Controller/Cardiovascular System/TPR Change/Venous Circ Vusv ==
  fes : Inport
  Gas(SI) : Inport  Port=2
  Constant : Constant  Value=ftas_min
  Constant1 : Constant  Value=initx(5)
  Divide : Product  Inputs=**
  Gain_Vusv : Gain  Gain=-265.4  SaturateOnIntegerOverflow=on  OutDataTypeStr=Inherit: Same as input  ParamDataTypeStr=Inherit: Same as input
  Math Function : Math  Operator=log  SaturateOnIntegerOverflow=on
  Saturation : Saturate  UpperLimit=inf  LowerLimit=1
  Sum : Sum  Inputs=|+-  SaturateOnIntegerOverflow=on  InputSameDT=on  OutDataTypeStr=Inherit: Same as first input
  Sum1 : Sum  SaturateOnIntegerOverflow=on  InputSameDT=on  OutDataTypeStr=Inherit: Same as first input
  Transfer Fcn : TransferFcn  Denominator=[toux(5)*0.7 1]
  Transport Delay : TransportDelay  DelayTime=Dx(5)*0.7  InitialOutput=10  BufferSize=19456
  Vusv : Outport
  wires:
  fes/1 -> Transport Delay/1
  Transport Delay/1 -> Sum/1
  Constant/1 -> Sum/2
  Sum/1 -> Saturation/1
  Saturation/1 -> Math Function/1
  Math Function/1 -> Gain_Vusv/1
  Transfer Fcn/1 -> Sum1/1
  Sum1/1 -> Vusv/1
  Constant1/1 -> Sum1/2
  Gas(SI)/1 -> Divide/2
  Gain_Vusv/1 -> Divide/1
  Divide/1 -> Transfer Fcn/1

== system Ventilator_Controller/Central Neural Control/Saving AutonomicCtrl/Switch Case Action Subsystem ==
  In1 : Inport
  Action Port : ActionPort  ActionPortLabel=case [ 0 ]:
  To File : ToFile  Filename=AutonomicCtrl1.mat  MatrixName=ftas_ftbs_ftp  SampleTime=sampletime
  wires:
  In1/1 -> To File/1

== system Ventilator_Controller/Central Neural Control/Saving AutonomicCtrl/Switch Case Action Subsystem1 ==
  In1 : Inport
  Action Port : ActionPort  ActionPortLabel=case [ 1 ]:
  To File : ToFile  Filename=AutonomicCtrl2.mat  MatrixName=ftas_ftbs_ftp  SampleTime=sampletime
  wires:
  In1/1 -> To File/1

== system Ventilator_Controller/Central Neural Control/Saving AutonomicCtrl/Switch Case Action Subsystem2 ==
  In1 : Inport
  Action Port : ActionPort  ActionPortLabel=case [ 2 ]:
  To File : ToFile  Filename=AutonomicCtrl3.mat  MatrixName=ftas_ftbs_ftp  SampleTime=sampletime
  wires:
  In1/1 -> To File/1

== system Ventilator_Controller/Central Neural Control/Saving AutonomicCtrl/Switch Case Action Subsystem3 ==
  In1 : Inport
  Action Port : ActionPort  ActionPortLabel=default:
  To File : ToFile  Filename=AutonomicCtrl10.mat  MatrixName=ftas_ftbs_ftp  SampleTime=sampletime
  wires:
  In1/1 -> To File/1

== system Ventilator_Controller/Central Neural Control/Saving AutonomicCtrl/Switch Case Action Subsystem4 ==
  In1 : Inport
  Action Port : ActionPort  ActionPortLabel=case [ 3 ]:
  To File : ToFile  Filename=AutonomicCtrl4.mat  MatrixName=ftas_ftbs_ftp  SampleTime=sampletime
  wires:
  In1/1 -> To File/1

== system Ventilator_Controller/Central Neural Control/Saving AutonomicCtrl/Switch Case Action Subsystem5 ==
  In1 : Inport
  Action Port : ActionPort  ActionPortLabel=case [ 4 ]:
  To File : ToFile  Filename=AutonomicCtrl5.mat  MatrixName=ftas_ftbs_ftp  SampleTime=sampletime
  wires:
  In1/1 -> To File/1

== system Ventilator_Controller/Central Neural Control/Saving AutonomicCtrl/Switch Case Action Subsystem6 ==
  In1 : Inport
  Action Port : ActionPort  ActionPortLabel=case [ 5 ]:
  To File : ToFile  Filename=AutonomicCtrl6.mat  MatrixName=ftas_ftbs_ftp  SampleTime=sampletime
  wires:
  In1/1 -> To File/1

== system Ventilator_Controller/Central Neural Control/Saving AutonomicCtrl/Switch Case Action Subsystem7 ==
  In1 : Inport
  Action Port : ActionPort  ActionPortLabel=case [ 6 ]:
  To File : ToFile  Filename=AutonomicCtrl7.mat  MatrixName=ftas_ftbs_ftp  SampleTime=sampletime
  wires:
  In1/1 -> To File/1

== system Ventilator_Controller/Central Neural Control/Saving AutonomicCtrl/Switch Case Action Subsystem8 ==
  In1 : Inport
  Action Port : ActionPort  ActionPortLabel=case [ 7 ]:
  To File : ToFile  Filename=AutonomicCtrl8.mat  MatrixName=ftas_ftbs_ftp  SampleTime=sampletime
  wires:
  In1/1 -> To File/1

== system Ventilator_Controller/Central Neural Control/Saving AutonomicCtrl/Switch Case Action Subsystem9 ==
  In1 : Inport
  Action Port : ActionPort  ActionPortLabel=case [ 8 ]:
  To File : ToFile  Filename=AutonomicCtrl9.mat  MatrixName=ftas_ftbs_ftp  SampleTime=sampletime
  wires:
  In1/1 -> To File/1

== system Ventilator_Controller/Central Neural Control/Saving Nt/Switch Case Action Subsystem ==
  In1 : Inport
  Action Port : ActionPort  ActionPortLabel=case [ 0 ]:
  To File : ToFile  Filename=Nt1.mat  MatrixName=Nt  SampleTime=sampletime
  wires:
  In1/1 -> To File/1

== system Ventilator_Controller/Central Neural Control/Saving Nt/Switch Case Action Subsystem1 ==
  In1 : Inport
  Action Port : ActionPort  ActionPortLabel=case [ 1 ]:
  To File : ToFile  Filename=Nt2.mat  MatrixName=Nt  SampleTime=sampletime
  wires:
  In1/1 -> To File/1

== system Ventilator_Controller/Central Neural Control/Saving Nt/Switch Case Action Subsystem2 ==
  In1 : Inport
  Action Port : ActionPort  ActionPortLabel=case [ 2 ]:
  To File : ToFile  Filename=Nt3.mat  MatrixName=Nt  SampleTime=sampletime
  wires:
  In1/1 -> To File/1

== system Ventilator_Controller/Central Neural Control/Saving Nt/Switch Case Action Subsystem3 ==
  In1 : Inport
  Action Port : ActionPort  ActionPortLabel=default:
  To File : ToFile  Filename=Nt10.mat  MatrixName=Nt  SampleTime=sampletime
  wires:
  In1/1 -> To File/1

== system Ventilator_Controller/Central Neural Control/Saving Nt/Switch Case Action Subsystem4 ==
  In1 : Inport
  Action Port : ActionPort  ActionPortLabel=case [ 3 ]:
  To File : ToFile  Filename=Nt4.mat  MatrixName=Nt  SampleTime=sampletime
  wires:
  In1/1 -> To File/1

== system Ventilator_Controller/Central Neural Control/Saving Nt/Switch Case Action Subsystem5 ==
  In1 : Inport
  Action Port : ActionPort  ActionPortLabel=case [ 4 ]:
  To File : ToFile  Filename=Nt5.mat  MatrixName=Nt  SampleTime=sampletime
  wires:
  In1/1 -> To File/1

== system Ventilator_Controller/Central Neural Control/Saving Nt/Switch Case Action Subsystem6 ==
  In1 : Inport
  Action Port : ActionPort  ActionPortLabel=case [ 5 ]:
  To File : ToFile  Filename=Nt6.mat  MatrixName=Nt  SampleTime=sampletime
  wires:
  In1/1 -> To File/1

== system Ventilator_Controller/Central Neural Control/Saving Nt/Switch Case Action Subsystem7 ==
  In1 : Inport
  Action Port : ActionPort  ActionPortLabel=case [ 6 ]:
  To File : ToFile  Filename=Nt7.mat  MatrixName=Nt  SampleTime=sampletime
  wires:
  In1/1 -> To File/1

== system Ventilator_Controller/Central Neural Control/Saving Nt/Switch Case Action Subsystem8 ==
  In1 : Inport
  Action Port : ActionPort  ActionPortLabel=case [ 7 ]:
  To File : ToFile  Filename=Nt8.mat  MatrixName=Nt  SampleTime=sampletime
  wires:
  In1/1 -> To File/1

== system Ventilator_Controller/Central Neural Control/Saving Nt/Switch Case Action Subsystem9 ==
  In1 : Inport
  Action Port : ActionPort  ActionPortLabel=case [ 8 ]:
  To File : ToFile  Filename=Nt9.mat  MatrixName=Nt  SampleTime=sampletime
  wires:
  In1/1 -> To File/1

== system Ventilator_Controller/Central Neural Control/Saving Resp_Rhythm/Switch Case Action Subsystem ==
  In1 : Inport
  Action Port : ActionPort  ActionPortLabel=case [ 0 ]:
  To File : ToFile  Filename=Resp_Rhythm1.mat  MatrixName=Resp_Rhythm  SampleTime=sampletime
  wires:
  In1/1 -> To File/1

== system Ventilator_Controller/Central Neural Control/Saving Resp_Rhythm/Switch Case Action Subsystem1 ==
  In1 : Inport
  Action Port : ActionPort  ActionPortLabel=case [ 1 ]:
  To File : ToFile  Filename=Resp_Rhythm2.mat  MatrixName=Resp_Rhythm  SampleTime=sampletime
  wires:
  In1/1 -> To File/1

== system Ventilator_Controller/Central Neural Control/Saving Resp_Rhythm/Switch Case Action Subsystem2 ==
  In1 : Inport
  Action Port : ActionPort  ActionPortLabel=case [ 2 ]:
  To File : ToFile  Filename=Resp_Rhythm3.mat  MatrixName=Resp_Rhythm  SampleTime=sampletime
  wires:
  In1/1 -> To File/1

== system Ventilator_Controller/Central Neural Control/Saving Resp_Rhythm/Switch Case Action Subsystem3 ==
  In1 : Inport
  Action Port : ActionPort  ActionPortLabel=default:
  To File : ToFile  Filename=Resp_Rhythm10.mat  MatrixName=Resp_Rhythm  SampleTime=sampletime
  wires:
  In1/1 -> To File/1

== system Ventilator_Controller/Central Neural Control/Saving Resp_Rhythm/Switch Case Action Subsystem4 ==
  In1 : Inport
  Action Port : ActionPort  ActionPortLabel=case [ 3 ]:
  To File : ToFile  Filename=Resp_Rhythm4.mat  MatrixName=Resp_Rhythm  SampleTime=sampletime
  wires:
  In1/1 -> To File/1

== system Ventilator_Controller/Central Neural Control/Saving Resp_Rhythm/Switch Case Action Subsystem5 ==
  In1 : Inport
  Action Port : ActionPort  ActionPortLabel=case [ 4 ]:
  To File : ToFile  Filename=Resp_Rhythm5.mat  MatrixName=Resp_Rhythm  SampleTime=sampletime
  wires:
  In1/1 -> To File/1

== system Ventilator_Controller/Central Neural Control/Saving Resp_Rhythm/Switch Case Action Subsystem6 ==
  In1 : Inport
  Action Port : ActionPort  ActionPortLabel=case [ 5 ]:
  To File : ToFile  Filename=Resp_Rhythm6.mat  MatrixName=Resp_Rhythm  SampleTime=sampletime
  wires:
  In1/1 -> To File/1

== system Ventilator_Controller/Central Neural Control/Saving Resp_Rhythm/Switch Case Action Subsystem7 ==
  In1 : Inport
  Action Port : ActionPort  ActionPortLabel=case [ 6 ]:
  To File : ToFile  Filename=Resp_Rhythm7.mat  MatrixName=Resp_Rhythm  SampleTime=sampletime
  wires:
  In1/1 -> To File/1

== system Ventilator_Controller/Central Neural Control/Saving Resp_Rhythm/Switch Case Action Subsystem8 ==
  In1 : Inport
  Action Port : ActionPort  ActionPortLabel=case [ 7 ]:
  To File : ToFile  Filename=Resp_Rhythm8.mat  MatrixName=Resp_Rhythm  SampleTime=sampletime
  wires:
  In1/1 -> To File/1

== system Ventilator_Controller/Central Neural Control/Saving Resp_Rhythm/Switch Case Action Subsystem9 ==
  In1 : Inport
  Action Port : ActionPort  ActionPortLabel=case [ 8 ]:
  To File : ToFile  Filename=Resp_Rhythm9.mat  MatrixName=Resp_Rhythm  SampleTime=sampletime
  wires:
  In1/1 -> To File/1

== system Ventilator_Controller/Central Neural Control/VARIABLE RESPIRATORY RHYTHM1/Enable Breathing Signal ==
  note: Original Logic is wrong! Changed Fcn1 and Fcn
  Enable Breathing : Inport
  Fcn : Fcn  Expr=(u(1)>0) * (1 ) + (u(1) <=0) * u(2)
  Fcn1 : Fcn  Expr=1-u
  Fcn2 : Fcn  Expr=(u(1)==0)*1+(u(1)==1)*u(2)
  Fcn3 : Fcn  Expr=(u(1)==0)*1+(u(1)==1)*u(2)
  Fcn4 : Fcn  Expr=(u(1)==0)*1+(u(1)==1)*u(2)
  Mux{,1..3} (4 alike) : Mux  Inputs=2
  Product1 : Product  Inputs=***  SaturateOnIntegerOverflow=on  InputSameDT=on  OutDataTypeStr=Inherit: Same as first input
  Enable_Breathing_Period : Outport
  wires:
  [Mueller_duration] -> Mux3/2
  [Mueller_activation] -> Mux3/1
  Mux3/1 -> Fcn2/1
  [Valsalva_activation] -> Mux1/1
  [Valsalva_duration] -> Mux1/2
  Mux1/1 -> Fcn3/1
  Fcn2/1 -> Product1/1
  Fcn3/1 -> Product1/2
  Product1/1 -> Fcn1/1
  Enable Breathing/1 -> Mux/2
  Mux/1 -> Fcn/1
  Fcn1/1 -> Mux/1
  Fcn/1 -> Enable_Breathing_Period/1
  Mux2/1 -> Fcn4/1
  Fcn4/1 -> Product1/3
  [FVC_activation] -> Mux2/1
  [FVC_duration] -> Mux2/2

== system Ventilator_Controller/Central Neural Control/VARIABLE RESPIRATORY RHYTHM1/Respiratory Rhythm_Generator ==
  VBP Variable Breathing Period : Inport
  Enable : EnablePort  StatesWhenEnabling=reset
  Constant : Constant
  Gain : Gain  Gain=0.5  SaturateOnIntegerOverflow=on  OutDataTypeStr=Inherit: Same as input  ParamDataTypeStr=Inherit: Same as input
  Inspiration<Expiration : Gain  Gain=1.5/4  SaturateOnIntegerOverflow=on  OutDataTypeStr=Inherit: Same as input  ParamDataTypeStr=Inherit: Same as input
  Integrator : Integrator
  Sign : Signum  ZeroCross=off
  Sum : Sum  Inputs=|+-  SaturateOnIntegerOverflow=on
  Sum1 : Sum  SaturateOnIntegerOverflow=on
  Respiratory Rhythm : Outport  InitialOutput=1.2221e-017
  wires:
  Constant/1 -> Integrator/1, Sum1/2
  Integrator/1 -> Sum/2
  Sum/1 -> Sign/1
  Sum1/1 -> Gain/1
  Sign/1 -> Sum1/1
  Gain/1 -> Respiratory Rhythm/1
  VBP Variable Breathing Period/1 -> Inspiration<Expiration/1
  Inspiration<Expiration/1 -> Sum/1

== system Ventilator_Controller/Central Neural Control/VARIABLE RESPIRATORY RHYTHM1/Variable Breathing Period Reset ==
  note: Variable Breathing Period Reset
  Breathing Freq (breaths/min) : Inport
  Abs : Abs  SaturateOnIntegerOverflow=on
  Abs1 : Abs  SaturateOnIntegerOverflow=on
  Constant : Constant
  Constant1 : Constant  Value=-1
  Derivative : Derivative
  If : If  IfExpression=u1 <0  ShowElse=off
  If Action Subsystem : Subsystem  TreatAsAtomicUnit=on
  Integrator : Integrator  ExternalReset=rising
  Integrator1 : Integrator  ExternalReset=rising
  Memory : Memory
  Mux : Mux  Inputs=3
  S_wake3 : Gain  Gain=1/60  SaturateOnIntegerOverflow=on  OutDataTypeStr=Inherit: Same as input  ParamDataTypeStr=Inherit: Same as input
  Saving BreathingPeriod : Subsystem
  Sign : Signum
  Sum : Sum  Inputs=|+-  SaturateOnIntegerOverflow=on
  Sum1 : Sum  Inputs=|++  SaturateOnIntegerOverflow=on
  Enable Breathing Signal : Outport
  Variable Breathing Period : Outport  Port=2
  wires:
  Breathing Freq (breaths/min)/1 -> S_wake3/1
  Integrator/1 -> Sum/2
  Sign/1 -> Abs/1
  Abs/1 -> Sum1/1, Memory/1
  Constant1/1 -> Sum1/2
  Memory/1 -> Integrator/2, Integrator1/2
  Sum1/1 -> Abs1/1
  Abs1/1 -> Enable Breathing Signal/1
  Derivative/1 -> Sign/1
  Sum/1 -> If/1, Mux/1  "BPin"
  Mux/1 -> Saving BreathingPeriod/1(In1)
  Constant/1 -> Integrator1/1, Sum/1
  Integrator1/1 -> If Action Subsystem/1(In1)
  If Action Subsystem/1(Out1) -> Mux/3, Derivative/1, Variable Breathing Period/1
  If/1 -> If Action Subsystem/Action
  S_wake3/1 -> Integrator/1, Mux/2
